simulink model "ExCount_naive_model"  (R2019b)
settings: Solver=ode45  StartTime=0.0  StopTime=100e-6  RelTol=1e-3  EnableMultiTasking=on
values from neighbouring files (symbols this model uses):
  fsig = 13.0e3    (= 13000)    [ExCount.m]
  M = OSR    (= 16)    [ExCount.m]
  OSR = 16    [ExCount.m]
  tclk = Ts    (= 6.25e-07)    [ExCount.m]
  vfs = vref*2    (= 1.8)    [ExCount.m]
  vin_amp = 10.^(vin_amp_dB/20)*vref    [ExCount.m]
  vref = 0.9    [ExCount.m]
settings Model: Creator=chench  LastModifiedBy=benve
settings DataIOCC: LimitDataPoints=on  SaveFormat=Array  ReturnWorkspaceOutputs=off
settings OptimizationCC: ExpressionDepthLimit=2147483647  InitFltsAndDblsToZero=on  LifeSpan=inf
settings DebuggingCC: SaveWithParameterizedLinksMsg=none  UnderspecifiedInitializationDetection=Classic  MergeDetectMultiDrivingBlocksExec=none  SignalResolutionControl=TryResolveAllWithWarning  SolverPrmCheckMsg=warning  MultiTaskDSMMsg=warning  MultiTaskCondExecSysMsg=none  FcnCallInpInsideContextMsg=warning  AllowSymbolicDim=off  StateNameClashWarn=warning  SFUnexpectedBacktrackingDiag=warning  SFNoUnconditionalDefaultTransitionDiag=warning  SFExecutionAtInitializationDiag=none  ArithmeticOperatorsInVariantConditions=warning
settings HardwareCC: ProdBitPerPointer=32  ProdBitPerSizeT=32  ProdBitPerPtrDiffT=32  ProdLargestAtomicFloat=None  ProdIntDivRoundTo=Undefined  ProdEndianess=Unspecified  ProdWordSize=32  ProdHWDeviceType=32-bit Generic
settings ModelReferenceCC: PropagateSignalLabelsOutOfModel=off
settings SFSimCC: SimUseLocalCustomCode=off  CustomCodeUndefinedFunction=UseInterfaceOnly
settings RTWCC: RTWUseLocalCustomCode=off
settings CodeAppCC: StateflowObjectComments=on
settings GRTTargetCC: TargetFcnLib=ansi_tfl_tmw.mat  TargetLangStandard=C89/C90 (ANSI)  GeneratePreprocessorConditionals=Disable all  CombineOutputUpdateFcns=off  GRTInterface=on
settings ConfigComp: CovMetricSettings=dw  CovHtmlReporting=on  CovSaveCumulativeToWorkspaceVar=on  CovSaveSingleToWorkspaceVar=on  CovExternalEMLEnable=off

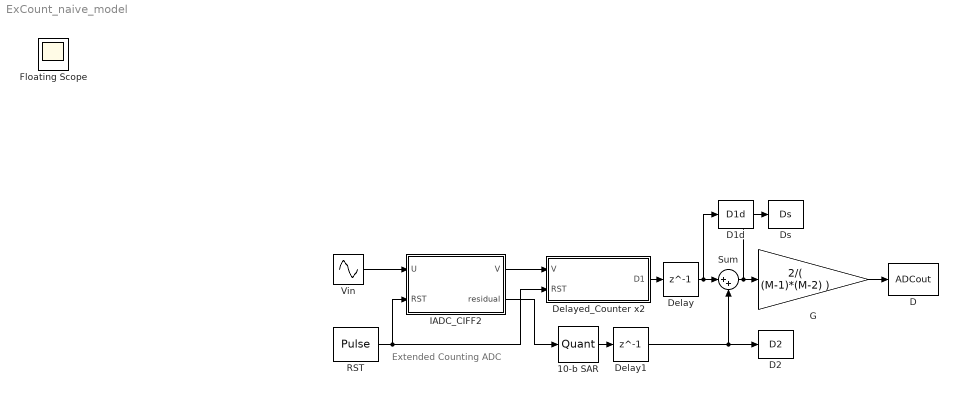
== system ExCount_naive_model ==
  note: Extended Counting ADC
  10-b SAR : Quantizer  QuantizationInterval=vfs/1024  LinearizeAsGain=off
  D : ToWorkspace  VariableName=ADCout  SampleTime=-1
  D1d : ToWorkspace  VariableName=D1d  SampleTime=-1
  D2 : ToWorkspace  VariableName=D2  SampleTime=-1
  Delay : Delay  DelayLength=1  InitialCondition=0
  Delay1 : Delay  DelayLength=1  InitialCondition=0
  Delayed_Counter x2 : Subsystem
  Ds : ToWorkspace  VariableName=Ds  SampleTime=-1
  G : Gain  Gain=2/( (M-1)*(M-2) )
  IADC_CIFF2 : Subsystem
  RST : DiscretePulseGenerator  Period=OSR  SampleTime=tclk
  Sum : Sum  Inputs=|++
  Vin : Sin  Amplitude=vin_amp  Frequency=fsig*2*pi  SampleTime=tclk
  Floating Scope : Scope
  wires:
  Sum/1 -> Ds/1, G/1
  RST/1 -> IADC_CIFF2/2(RST), Delayed_Counter x2/2(RST)
  G/1 -> D/1
  IADC_CIFF2/2(residual) -> 10-b SAR/1
  Delayed_Counter x2/1(D1) -> Delay/1
  Vin/1 -> IADC_CIFF2/1(U)
  IADC_CIFF2/1(V) -> Delayed_Counter x2/1(V)
  Delay/1 -> D1d/1, Sum/1
  10-b SAR/1 -> Delay1/1
  Delay1/1 -> Sum/2, D2/1

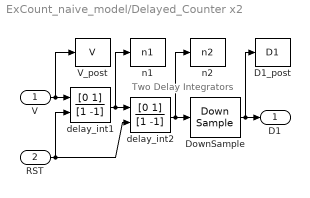
== system ExCount_naive_model/Delayed_Counter x2 ==
  note: Two Delay Integrators
  V : Inport
  RST : Inport  Port=2
  D1_post : ToWorkspace  VariableName=D1  SampleTime=-1
  DownSample : DownSample  N=OSR  phase=OSR-1  RateOptions=Allow multirate processing
  V_post : ToWorkspace  VariableName=V  SampleTime=-1
  delay_int1 : DiscreteFilter  Numerator=[0 1]  Denominator=[1 -1]  ExternalReset=Rising
      settings: InputPortMap=u0,r7
  delay_int2 : DiscreteFilter  Numerator=[0 1]  Denominator=[1 -1]  ExternalReset=Rising
      settings: InputPortMap=u0,r7
  n1 : ToWorkspace  VariableName=n1  SampleTime=-1
  n2 : ToWorkspace  VariableName=n2  SampleTime=-1
  D1 : Outport  VectorParamsAs1DForOutWhenUnconnected=off
  wires:
  delay_int1/1 -> n1/1, delay_int2/1
  V/1 -> V_post/1, delay_int1/1
  delay_int2/1 -> n2/1, DownSample/1
  RST/1 -> delay_int1/2, delay_int2/2
  DownSample/1 -> D1_post/1, D1/1

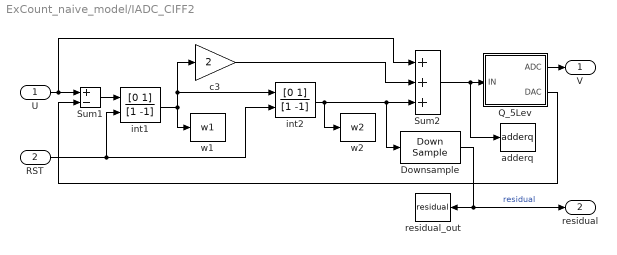
== system ExCount_naive_model/IADC_CIFF2 ==
  U : Inport
  RST : Inport  Port=2
  Downsample : DownSample  N=OSR  phase=OSR-1  RateOptions=Allow multirate processing
  Q_5Lev : Subsystem
  Sum1 : Sum  Inputs=+-  SaturateOnIntegerOverflow=on  InputSameDT=on  OutDataTypeStr=Inherit: Same as first input
  Sum2 : Sum  Inputs=+++  SaturateOnIntegerOverflow=on  InputSameDT=on  OutDataTypeStr=Inherit: Same as first input
  adderq : ToWorkspace  VariableName=adderq  SampleTime=-1
  c3 : Gain  Gain=2  SaturateOnIntegerOverflow=on  OutDataTypeStr=Inherit: Same as input  ParamDataTypeStr=Inherit: Same as input
  int1 : DiscreteFilter  Numerator=[0 1]  Denominator=[1 -1]  ExternalReset=Rising
      settings: InputPortMap=u0,r7
  int2 : DiscreteFilter  Numerator=[0 1]  Denominator=[1 -1]  ExternalReset=Rising
      settings: InputPortMap=u0,r7
  residual_out : ToWorkspace  VariableName=residual  SampleTime=-1
  w1 : ToWorkspace  VariableName=w1  SampleTime=-1
  w2 : ToWorkspace  VariableName=w2  SampleTime=-1
  V : Outport  VectorParamsAs1DForOutWhenUnconnected=off
  residual : Outport  Port=2  VectorParamsAs1DForOutWhenUnconnected=off
  wires:
  c3/1 -> Sum2/2
  Sum2/1 -> adderq/1, Q_5Lev/1(IN)
  int2/1 -> Sum2/3, Downsample/1, w2/1
  Q_5Lev/1(ADC) -> V/1
  Q_5Lev/2(DAC) -> Sum1/2
  Sum1/1 -> int1/1
  U/1 -> Sum2/1, Sum1/1
  Downsample/1 -> residual/1, residual_out/1  "residual"
  RST/1 -> int2/2, int1/2
  int1/1 -> w1/1, int2/1, c3/1

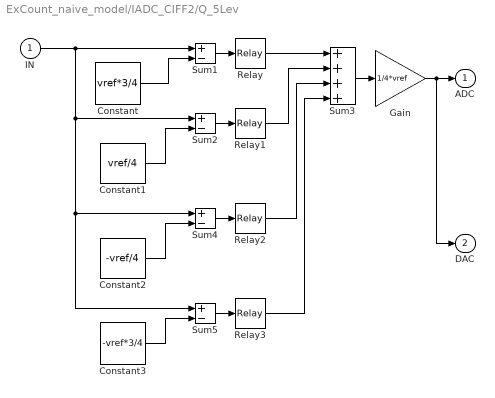
== system ExCount_naive_model/IADC_CIFF2/Q_5Lev ==
  IN : Inport
  Constant : Constant  Value=vref*3/4
  Constant1 : Constant  Value=vref/4
  Constant2 : Constant  Value=-vref/4
  Constant3 : Constant  Value=-vref*3/4
  Gain : Gain  Gain=1/4*vref
  Relay{,1..3} (4 alike) : Relay  OffOutputValue=-1  SampleTime=tclk
  Sum{1..2,4..5} (4 alike) : Sum  Inputs=+-  SaturateOnIntegerOverflow=on  InputSameDT=on  OutDataTypeStr=Inherit: Same as first input
  Sum3 : Sum  Inputs=++++  SaturateOnIntegerOverflow=on  InputSameDT=on  OutDataTypeStr=Inherit: Same as first input
  ADC : Outport  VectorParamsAs1DForOutWhenUnconnected=off
  DAC : Outport  Port=2  VectorParamsAs1DForOutWhenUnconnected=off
  wires:
  Sum1/1 -> Relay/1
  Sum2/1 -> Relay1/1
  IN/1 -> Sum1/1, Sum2/1, Sum4/1, Sum5/1
  Constant/1 -> Sum1/2
  Constant1/1 -> Sum2/2
  Relay/1 -> Sum3/1
  Relay1/1 -> Sum3/2
  Sum3/1 -> Gain/1
  Sum4/1 -> Relay2/1
  Constant2/1 -> Sum4/2
  Relay2/1 -> Sum3/3
  Sum5/1 -> Relay3/1
  Constant3/1 -> Sum5/2
  Relay3/1 -> Sum3/4
  Gain/1 -> DAC/1, ADC/1
